simulink model "ObservadorPlantaRealCompatible"  (Simulink 7.9)
settings: Solver=ode3  SolverMode=SingleTasking  StartTime=0.0  StopTime=20  RelTol=1e-3
libraries: arduino_io_lib x5
settings Model: FPTRunName=Active  Creator=The MathWorks, Inc.  LastModifiedBy=i95sa  CovModelRefEnable=off  ExtModeTrigDuration=2
settings DataIOCC: SignalLoggingSaveFormat=Dataset
settings OptimizationCC: InlineParams=on  OptimizeModelRefInitCode=on  LifeSpan=Inf  MaxStackSize=64
settings DebuggingCC: SolverPrmCheckMsg=none  ParameterOverflowMsg=warning  FrameProcessingCompatibilityMsg=error
settings HardwareCC: ProdBitPerPointer=64  ProdLargestAtomicFloat=Float  ProdIntDivRoundTo=Zero  ProdEndianess=LittleEndian  ProdHWDeviceType=Specified
settings RTWCC: SystemTargetFile=ert.tlc  TemplateMakefile=ert_default_tmf  Description=Embedded Coder  GenerateReport=on  RTWVerbose=off  LaunchReport=on
settings CodeAppCC: ForceParamTrailComments=on  IgnoreCustomStorageClasses=off  SimulinkDataObjDesc=on  SFDataObjDesc=on  MATLABFcnDesc=on  InsertBlockDesc=on  MATLABSourceComments=on
settings ERTTargetCC: CodeReplacementLibrary=C89/C90 (ANSI)  MultiwordLength=2048  SupportNonInlinedSFcns=on  ERTCustomFileTemplate=example_file_process.tlc

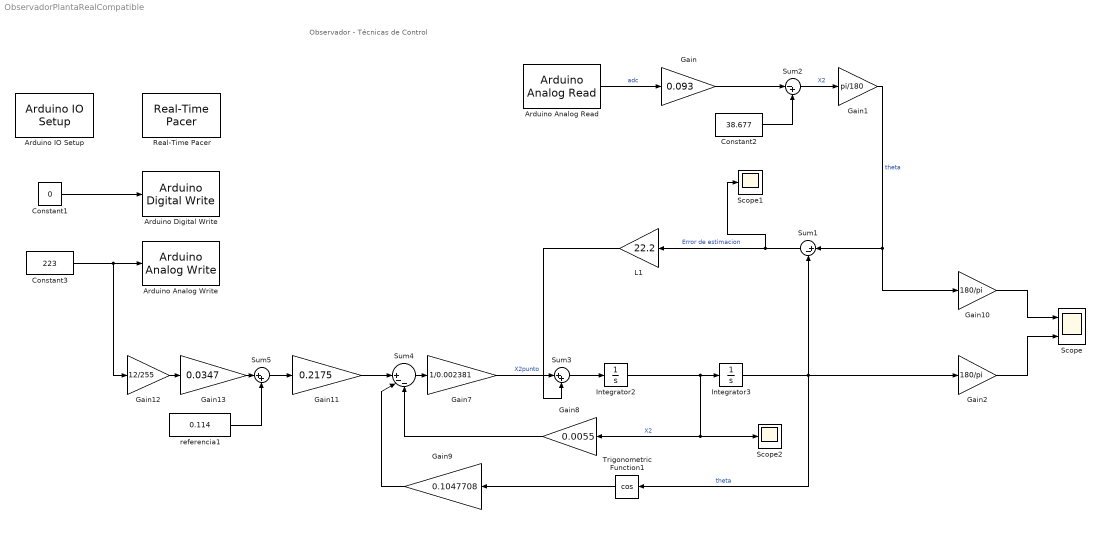
== system ObservadorPlantaRealCompatible ==
  note: Observador - Técnicas de Control
  Arduino Analog Read : arduino_io_lib/Arduino Analog Read  arduinoVar=Existing workspace arduino variable #1  arduinoPin=0  T=0.1
  Arduino Analog Write : arduino_io_lib/Arduino Analog Write  arduinoVar=Existing workspace arduino variable #1  arduinoPin=7  T=0.1
  Arduino Digital Write : arduino_io_lib/Arduino Digital Write  arduinoVar=Existing workspace arduino variable #1  arduinoPin=6  T=0.1
  Arduino IO Setup : arduino_io_lib/Arduino IO Setup  Priority=3  arduinoVar=Existing workspace arduino variable #1  workspaceVarName=a  comPort=4
  Constant1 : Constant  Value=0
  Constant2 : Constant  Value=38.677
  Constant3 : Constant  Value=223
  Gain : Gain  Gain=0.093
  Gain1 : Gain  Gain=pi/180
  Gain10 : Gain  Gain=180/pi
  Gain11 : Gain  Gain=0.2175
  Gain12 : Gain  Gain=12/255
  Gain13 : Gain  Gain=0.0347
  Gain2 : Gain  Gain=180/pi
  Gain7 : Gain  Gain=1/0.002381
  Gain8 : Gain  Gain=0.0055
  Gain9 : Gain  Gain=0.1047708
  Integrator2 : Integrator
  Integrator3 : Integrator  InitialCondition=-0.65
  L1 : Gain  Gain=22.2
  Real-Time Pacer : arduino_io_lib/Real-Time Pacer  simTimePerRealTime=1
  Scope : Scope  NumInputPorts=2
      settings: TimeRange=auto  MaxDataPoints=5000  SaveName=PosicionReal  YMin=-41.47638~-72.1356  YMax=26.29738~276.7978  SampleTime=-1
  Scope1 : Scope
      settings: TimeRange=auto  LimitDataPoints=on  MaxDataPoints=5000  SaveToWorkspace=off  YMin=-10  YMax=10  SampleTime=-1  DataFormat=Array
  Scope2 : Scope
      settings: TimeRange=auto  MaxDataPoints=5000  SaveName=VelocidadEstimada  YMin=-0.95376  YMax=1.30426  SampleTime=-1  DataFormat=Array
  Sum1 : Sum  Inputs=|+-
  Sum2 : Sum  Inputs=|-+
  Sum3 : Sum  Inputs=|++
  Sum4 : Sum  Inputs=||+--
  Sum5 : Sum  Inputs=|++
  Trigonometric Function1 : Trigonometry  Operator=cos
  referencia1 : Constant  Value=0.114
  wires:
  Arduino Analog Read/1 -> Gain/1  "adc"
  Constant1/1 -> Arduino Digital Write/1
  Gain/1 -> Sum2/1
  Constant2/1 -> Sum2/2
  Sum2/1 -> Gain1/1  "X2"
  Sum4/1 -> Gain7/1
  Trigonometric Function1/1 -> Gain9/1
  Gain8/1 -> Sum4/3
  Gain9/1 -> Sum4/2
  Gain11/1 -> Sum4/1
  referencia1/1 -> Sum5/2
  Sum5/1 -> Gain11/1
  Gain12/1 -> Gain13/1
  Gain13/1 -> Sum5/1
  Constant3/1 -> Arduino Analog Write/1, Gain12/1
  Gain2/1 -> Scope/2
  Gain10/1 -> Scope/1
  Gain1/1 -> Sum1/1, Gain10/1  "theta"
  Integrator3/1 -> Trigonometric Function1/1, Gain2/1, Sum1/2  "theta"
  Sum1/1 -> Scope1/1, L1/1  "Error de estimacion"
  Integrator2/1 -> Scope2/1, Gain8/1, Integrator3/1  "X2"
  Gain7/1 -> Sum3/1  "X2punto"
  L1/1 -> Sum3/2
  Sum3/1 -> Integrator2/1
